simulink model "decoupled_simulink"  (R2021b)
settings: Solver=VariableStepAuto  StartTime=0.0  StopTime=30  RelTol=1e-3
values from neighbouring files (symbols this model uses):
  B = [0, 0 ... (first row only)    [basic_data.m]    (also in basic_data.mat = [0  0; 0  0; 0  0; 27  11.2; 6.06660129535  -1.63757677119; ; lqr.mat = [0  0; 0  0; 0  0; 27  11.2; 6.06660129535  -1.63757677119; )
  C_2 = [1 0 0 0 0 0;0 0 1 0 0 0]    [decoupled.m]
  F = inv(B_star)    [decoupled.m]
settings Model: Creator=asus  LastModifiedBy=asus

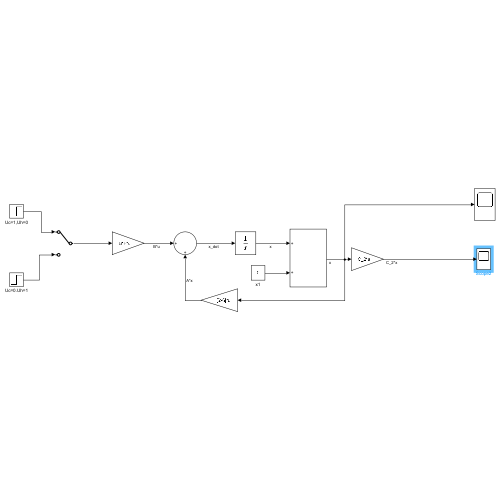
[thumbnail: Simulink's stored preview of the top-level diagram]
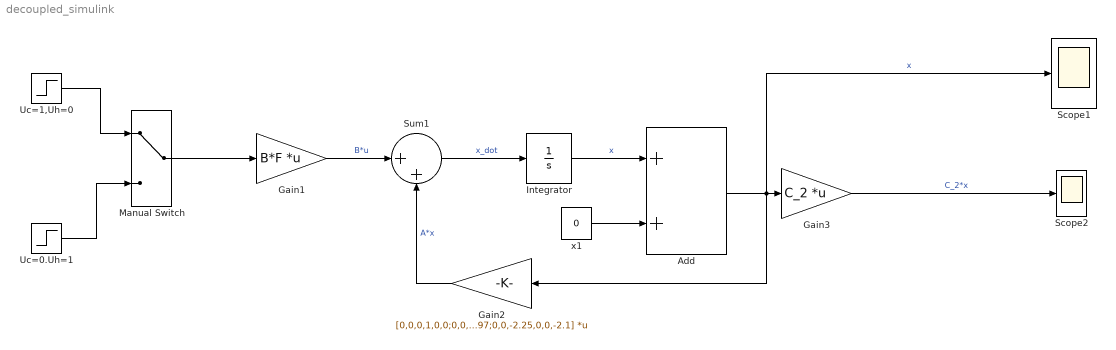
== system decoupled_simulink ==
  Add : Sum
  Gain1 : Gain  Gain=B*F  Multiplication=Matrix(K*u)
  Gain2 : Gain  Gain=[0,0,0,1,0,0;0,0,0,0,1,0;0,0,0,0,0,1;-2.25,0,0,-2.1,0,0;-22.3092,12.6549,14.5121,7.452,-4.4537,-3.4397;0,0,-2.25,0,0,-2.1]  Multiplication=Matrix(K*u)
  Gain3 : Gain  Gain=C_2  Multiplication=Matrix(K*u)
  Integrator : Integrator
  Manual Switch : ManualSwitch
  Scope1 : Scope
  Scope2 : Scope
  Sum1 : Sum  Inputs=|++
  Uc=0.Uh=1 : Step  Time=0  After=[0;1]  SampleTime=0
  Uc=1,Uh=0 : Step  Time=0  After=[1;0]  SampleTime=0
  x1 : Constant  Value=0  VectorParams1D=off
  wires:
  Integrator/1 -> Add/1  "x"
  Sum1/1 -> Integrator/1  "x_dot"
  Gain1/1 -> Sum1/1  "B*u"
  Gain2/1 -> Sum1/2  "A*x"
  Add/1 -> Gain2/1, Scope1/1, Gain3/1  "x"
  x1/1 -> Add/2
  Manual Switch/1 -> Gain1/1
  Uc=1,Uh=0/1 -> Manual Switch/1
  Uc=0.Uh=1/1 -> Manual Switch/2
  Gain3/1 -> Scope2/1  "C_2*x"
